simulink subsystem "Final_Project_DistHold_attempt_20260602_205044"  (R2024a)
settings: Solver=VariableStepAuto  StartTime=0.0  StopTime=10.0  RelTol=1e-3
values from neighbouring files (symbols this model uses):
  D = hypot(Ep(:,1)-Tp(:,1)',Ep(:,2)-Tp(:,2)')    [pp_compare_stage.m]    (also in pp_diag_path.m; pp_t09_clear.m = hypot(Ep(:,1)-Tperim(:,1)', Ep(:,2)-Tperim(:,2)'); pp_tune2.m)
undefined symbols (not defined in the file or in its folder): DiscIntNeverNeededParam, waypoint_const
libraries: CarMaker4SL x83, simulink x2
(part 3 of 5)

== matlab function Final_Project_DistHold_attempt_20260602_205044/Driving_Module_Ver.3_PSH/Subsystem/Traffic_Detector ==
  data: ego_state input Bus: EgoStateBus; lead_dist output double; lanes input Bus: ParsedLaneBus; traffic input; target_speed input double; ego_lane_id input int32; lead_speed output double; left_clear output boolean; right_clear output boolean
function [lead_dist, lead_speed, left_clear, right_clear] = Traffic_Detector(ego_state, lanes, traffic, target_speed, ego_lane_id)
%#codegen
% traffic : Obstacle_Info_Bus
% 내부 구조 예:
%   traffic.t16.x, traffic.t16.y, traffic.t16.vx, traffic.t16.vy
%   ...
%   traffic.t28.x, traffic.t28.y, traffic.t28.vx, traffic.t28.vy
%
% 주의:
%   target_speed는 배선 호환용으로 남겨두지만, 거리 판단에는 ego_v를 사용함.

    unused_target_speed = target_speed; %#ok<NASGU>

    % ============================================================
    % 0. 출력 초기화
    % ============================================================
    lead_dist   = 1e9;
    lead_speed  = 0.0;
    left_clear  = true;
    right_clear = true;
    ego_lane    = int32(ego_lane_id);

    % ============================================================
    % 1. Ego unpack
    % ============================================================
    ego_x = ego_state.Car_Fr1_tx;
    ego_y = ego_state.Car_Fr1_ty;
    ego_v = ego_state.Ego_V;

    % ============================================================
    % 2. Lane unpack - 5차선
    % ============================================================
    x1 = lanes.x1; y1 = lanes.y1;
    x2 = lanes.x2; y2 = lanes.y2;
    x3 = lanes.x3; y3 = lanes.y3;
    x4 = lanes.x4; y4 = lanes.y4;
    x5 = lanes.x5; y5 = lanes.y5;

    % detector와 lane5 기준을 맞추기 위한 보정
    L5_OFFSET = 1.0;
    x5 = x5 + L5_OFFSET;

    % ============================================================
    % 3. Ego 속도 기반 가변 탐색/안전거리
    % ============================================================
    v_ego_gap = abs(ego_v);

    if v_ego_gap > 60.0
        v_ego_gap = v_ego_gap / 3.6;
    end

    LOOK_FRONT = calcLookFront(v_ego_gap);

    CLEAR_BACK_MIN = 5.0;
    CLEAR_BACK_TG  = 0.5;
    CLEAR_BACK_MAX = 35.0;

    CLEAR_BACK = CLEAR_BACK_MIN + CLEAR_BACK_TG * v_ego_gap;

    if CLEAR_BACK > CLEAR_BACK_MAX
        CLEAR_BACK = CLEAR_BACK_MAX;
    end

    CLEAR_FRONT_MIN = 15.0;
    CLEAR_FRONT_TG  = 0.9;
    CLEAR_FRONT_MAX = 70.0;

    CLEAR_FRONT = CLEAR_FRONT_MIN + CLEAR_FRONT_TG * v_ego_gap;

    if CLEAR_FRONT > CLEAR_FRONT_MAX
        CLEAR_FRONT = CLEAR_FRONT_MAX;
    end

    % ============================================================
    % 4. Init
    % ============================================================
    lead_dist  = 1e9;
    lead_speed = v_ego_gap;

    left_clear  = true;
    right_clear = true;

    if ego_lane >= int32(5)
        left_clear = false;
    end

    if ego_lane <= int32(1)
        right_clear = false;
    end

    % ============================================================
    % 5. Traffic_Info_16_Bus ~ Traffic_Info_28_Bus 직접 처리
    % ============================================================
    [lead_dist, lead_speed, left_clear, right_clear] = check_one_signal( ...
        traffic.t16.x, traffic.t16.y, traffic.t16.vx, traffic.t16.vy, true, ...
        ego_x, ego_y, ego_lane, ...
        x1,y1,x2,y2,x3,y3,x4,y4,x5,y5, ...
        lead_dist, lead_speed, left_clear, right_clear, ...
        LOOK_FRONT, CLEAR_BACK, CLEAR_FRONT);

    [lead_dist, lead_speed, left_clear, right_clear] = check_one_signal( ...
        traffic.t17.x, traffic.t17.y, traffic.t17.vx, traffic.t17.vy, true, ...
        ego_x, ego_y, ego_lane, ...
        x1,y1,x2,y2,x3,y3,x4,y4,x5,y5, ...
        lead_dist, lead_speed, left_clear, right_clear, ...
        LOOK_FRONT, CLEAR_BACK, CLEAR_FRONT);

    [lead_dist, lead_speed, left_clear, right_clear] = check_one_signal( ...
        traffic.t18.x, traffic.t18.y, traffic.t18.vx, traffic.t18.vy, true, ...
        ego_x, ego_y, ego_lane, ...
        x1,y1,x2,y2,x3,y3,x4,y4,x5,y5, ...
        lead_dist, lead_speed, left_clear, right_clear, ...
        LOOK_FRONT, CLEAR_BACK, CLEAR_FRONT);

    [lead_dist, lead_speed, left_clear, right_clear] = check_one_signal( ...
        traffic.t19.x, traffic.t19.y, traffic.t19.vx, traffic.t19.vy, true, ...
        ego_x, ego_y, ego_lane, ...
        x1,y1,x2,y2,x3,y3,x4,y4,x5,y5, ...
        lead_dist, lead_speed, left_clear, right_clear, ...
        LOOK_FRONT, CLEAR_BACK, CLEAR_FRONT);

    [lead_dist, lead_speed, left_clear, right_clear] = check_one_signal( ...
        traffic.t20.x, traffic.t20.y, traffic.t20.vx, traffic.t20.vy, true, ...
        ego_x, ego_y, ego_lane, ...
        x1,y1,x2,y2,x3,y3,x4,y4,x5,y5, ...
        lead_dist, lead_speed, left_clear, right_clear, ...
        LOOK_FRONT, CLEAR_BACK, CLEAR_FRONT);

    [lead_dist, lead_speed, left_clear, right_clear] = check_one_signal( ...
        traffic.t21.x, traffic.t21.y, traffic.t21.vx, traffic.t21.vy, true, ...
        ego_x, ego_y, ego_lane, ...
        x1,y1,x2,y2,x3,y3,x4,y4,x5,y5, ...
        lead_dist, lead_speed, left_clear, right_clear, ...
        LOOK_FRONT, CLEAR_BACK, CLEAR_FRONT);

    [lead_dist, lead_speed, left_clear, right_clear] = check_one_signal( ...
        traffic.t22.x, traffic.t22.y, traffic.t22.vx, traffic.t22.vy, true, ...
        ego_x, ego_y, ego_lane, ...
        x1,y1,x2,y2,x3,y3,x4,y4,x5,y5, ...
        lead_dist, lead_speed, left_clear, right_clear, ...
        LOOK_FRONT, CLEAR_BACK, CLEAR_FRONT);

    [lead_dist, lead_speed, left_clear, right_clear] = check_one_signal( ...
        traffic.t23.x, traffic.t23.y, traffic.t23.vx, traffic.t23.vy, true, ...
        ego_x, ego_y, ego_lane, ...
        x1,y1,x2,y2,x3,y3,x4,y4,x5,y5, ...
        lead_dist, lead_speed, left_clear, right_clear, ...
        LOOK_FRONT, CLEAR_BACK, CLEAR_FRONT);

    [lead_dist, lead_speed, left_clear, right_clear] = check_one_signal( ...
        traffic.t24.x, traffic.t24.y, traffic.t24.vx, traffic.t24.vy, true, ...
        ego_x, ego_y, ego_lane, ...
        x1,y1,x2,y2,x3,y3,x4,y4,x5,y5, ...
        lead_dist, lead_speed, left_clear, right_clear, ...
        LOOK_FRONT, CLEAR_BACK, CLEAR_FRONT);

    [lead_dist, lead_speed, left_clear, right_clear] = check_one_signal( ...
        traffic.t25.x, traffic.t25.y, traffic.t25.vx, traffic.t25.vy, true, ...
        ego_x, ego_y, ego_lane, ...
        x1,y1,x2,y2,x3,y3,x4,y4,x5,y5, ...
        lead_dist, lead_speed, left_clear, right_clear, ...
        LOOK_FRONT, CLEAR_BACK, CLEAR_FRONT);

    [lead_dist, lead_speed, left_clear, right_clear] = check_one_signal( ...
        traffic.t26.x, traffic.t26.y, traffic.t26.vx, traffic.t26.vy, true, ...
        ego_x, ego_y, ego_lane, ...
        x1,y1,x2,y2,x3,y3,x4,y4,x5,y5, ...
        lead_dist, lead_speed, left_clear, right_clear, ...
        LOOK_FRONT, CLEAR_BACK, CLEAR_FRONT);

    [lead_dist, lead_speed, left_clear, right_clear] = check_one_signal( ...
        traffic.t27.x, traffic.t27.y, traffic.t27.vx, traffic.t27.vy, true, ...
        ego_x, ego_y, ego_lane, ...
        x1,y1,x2,y2,x3,y3,x4,y4,x5,y5, ...
        lead_dist, lead_speed, left_clear, right_clear, ...
        LOOK_FRONT, CLEAR_BACK, CLEAR_FRONT);

    [lead_dist, lead_speed, left_clear, right_clear] = check_one_signal( ...
        traffic.t28.x, traffic.t28.y, traffic.t28.vx, traffic.t28.vy, true, ...
        ego_x, ego_y, ego_lane, ...
        x1,y1,x2,y2,x3,y3,x4,y4,x5,y5, ...
        lead_dist, lead_speed, left_clear, right_clear, ...
        LOOK_FRONT, CLEAR_BACK, CLEAR_FRONT);

end


function LOOK_FRONT = calcLookFront(v)
%#codegen
    v = abs(v);

    if v > 60.0
        v = v / 3.6;
    end

    V_HIGH = 80.0 / 3.6;

    if v < V_HIGH
        LOOK_FRONT = 25.0 + 1.0 * v;
    else
        LOOK_FRONT = 25.0 + 1.0 * V_HIGH + 10.0 * (v - V_HIGH);
    end

    if LOOK_FRONT > 120.0
        LOOK_FRONT = 120.0;
    end
end


function [lead_dist, lead_speed, left_clear, right_clear] = check_one_signal( ...
    obj_x, obj_y, obj_vx, obj_vy, valid, ...
    ego_x, ego_y, ego_lane_id, ...
    x1,y1,x2,y2,x3,y3,x4,y4,x5,y5, ...
    lead_dist, lead_speed, left_clear, right_clear, ...
    LOOK_FRONT, CLEAR_BACK, CLEAR_FRONT)
%#codegen

    if ~valid
        return;
    end

    [lead_dist, lead_speed, left_clear, right_clear] = check_one_vehicle( ...
        ego_x, ego_y, ego_lane_id, ...
        obj_x, obj_y, obj_vx, obj_vy, ...
        x1,y1,x2,y2,x3,y3,x4,y4,x5,y5, ...
        lead_dist, lead_speed, left_clear, right_clear, ...
        LOOK_FRONT, CLEAR_BACK, CLEAR_FRONT);

end


function [lead_dist, lead_speed, left_clear, right_clear] = check_one_vehicle( ...
    ego_x, ego_y, ego_lane_id, ...
    obj_x, obj_y, obj_vx, obj_vy, ...
    x1, y1, x2, y2, x3, y3, x4, y4, x5, y5, ...
    lead_dist, lead_speed, left_clear, right_clear, ...
    LOOK_FRONT, CLEAR_BACK, CLEAR_FRONT)
%#codegen

    [obj_lane_id, obj_idx] = nearest_lane_id( ...
        obj_x, obj_y, ...
        x1, y1, x2, y2, x3, y3, x4, y4, x5, y5);

    if obj_lane_id == ego_lane_id

        ego_idx = nearest_idx_by_lane( ...
            ego_lane_id, ego_x, ego_y, ...
            x1, y1, x2, y2, x3, y3, x4, y4, x5, y5);

        s_rel = arc_dist_forward_by_lane( ...
            ego_lane_id, ego_idx, obj_idx, ...
            x1, y1, x2, y2, x3, y3, x4, y4, x5, y5);

        if s_rel > 0.0 && s_rel < LOOK_FRONT
            if s_rel < lead_dist
                lead_dist  = s_rel;
                lead_speed = sqrt(obj_vx*obj_vx + obj_vy*obj_vy);
            end
        end
    end

    if obj_lane_id == ego_lane_id + int32(1)

        ego_idx_adj = nearest_idx_by_lane( ...
            obj_lane_id, ego_x, ego_y, ...
            x1, y1, x2, y2, x3, y3, x4, y4, x5, y5);

        is_close = is_close_on_adj_lane( ...
            obj_lane_id, ego_idx_adj, obj_idx, ...
            CLEAR_BACK, CLEAR_FRONT, ...
            x1, y1, x2, y2, x3, y3, x4, y4, x5, y5);

        if is_close
            left_clear = false;
        end

    elseif obj_lane_id == ego_lane_id - int32(1)

        ego_idx_adj = nearest_idx_by_lane( ...
            obj_lane_id, ego_x, ego_y, ...
            x1, y1, x2, y2, x3, y3, x4, y4, x5, y5);

        is_close = is_close_on_adj_lane( ...
            obj_lane_id, ego_idx_adj, obj_idx, ...
            CLEAR_BACK, CLEAR_FRONT, ...
            x1, y1, x2, y2, x3, y3, x4, y4, x5, y5);

        if is_close
            right_clear = false;
        end
    end

end


function [lane_id, best_idx] = nearest_lane_id(px, py, x1, y1, x2, y2, x3, y3, x4, y4, x5, y5)
%#codegen

    [idx1, d1] = nearest_idx_d2(x1, y1, px, py);
    [idx2, d2] = nearest_idx_d2(x2, y2, px, py);
    [idx3, d3] = nearest_idx_d2(x3, y3, px, py);
    [idx4, d4] = nearest_idx_d2(x4, y4, px, py);
    [idx5, d5] = nearest_idx_d2(x5, y5, px, py);

    lane_id  = int32(1);
    best_idx = idx1;
    best_d2  = d1;

    if d2 < best_d2
        lane_id  = int32(2);
        best_idx = idx2;
        best_d2  = d2;
    end

    if d3 < best_d2
        lane_id  = int32(3);
        best_idx = idx3;
        best_d2  = d3;
    end

    if d4 < best_d2
        lane_id  = int32(4);
        best_idx = idx4;
        best_d2  = d4;
    end

    if d5 < best_d2
        lane_id  = int32(5);
        best_idx = idx5;
    end

end


function idx = nearest_idx_by_lane(lane_id, px, py, x1, y1, x2, y2, x3, y3, x4, y4, x5, y5)
%#codegen

    if lane_id == int32(1)
        [idx, ~] = nearest_idx_d2(x1, y1, px, py);
    elseif lane_id == int32(2)
        [idx, ~] = nearest_idx_d2(x2, y2, px, py);
    elseif lane_id == int32(3)
        [idx, ~] = nearest_idx_d2(x3, y3, px, py);
    elseif lane_id == int32(4)
        [idx, ~] = nearest_idx_d2(x4, y4, px, py);
    else
        [idx, ~] = nearest_idx_d2(x5, y5, px, py);
    end

end


function [best_i, best_d2] = nearest_idx_d2(xa, ya, px, py)
%#codegen

    best_i  = int32(1);
    best_d2 = 1e12;
    N = int32(numel(xa));

    for i = 1:N
        dx = xa(i) - px;
        dy = ya(i) - py;
        d2 = dx*dx + dy*dy;

        if d2 < best_d2
            best_d2 = d2;
            best_i  = i;
        end
    end

end


function ds = arc_dist_forward_by_lane(lane_id, idx_from, idx_to, ...
    x1, y1, x2, y2, x3, y3, x4, y4, x5, y5)
%#codegen

    if lane_id == int32(1)
        ds = arc_dist_forward_closed(x1, y1, idx_from, idx_to);
    elseif lane_id == int32(2)
        ds = arc_dist_forward_closed(x2, y2, idx_from, idx_to);
    elseif lane_id == int32(3)
        ds = arc_dist_forward_closed(x3, y3, idx_from, idx_to);
    elseif lane_id == int32(4)
        ds = arc_dist_open(x4, y4, idx_from, idx_to);
    else
        ds = arc_dist_open(x5, y5, idx_from, idx_to);
    end

end


function ds = arc_dist_forward_closed(xa, ya, idx_from, idx_to)
%#codegen

    ds = 0.0;
    N = int32(numel(xa));

    if idx_to == idx_from
        ds = 0.0;
        return;
    end

    if idx_to > idx_from

        for i = idx_from:(idx_to - int32(1))
            dx = xa(i+1) - xa(i);
            dy = ya(i+1) - ya(i);
            ds = ds + sqrt(dx*dx + dy*dy);
        end

    else

        for i = idx_from:(N - int32(1))
            dx = xa(i+1) - xa(i);
            dy = ya(i+1) - ya(i);
            ds = ds + sqrt(dx*dx + dy*dy);
        end

        dx = xa(1) - xa(N);
        dy = ya(1) - ya(N);
        ds = ds + sqrt(dx*dx + dy*dy);

        for i = int32(1):(idx_to - int32(1))
            dx = xa(i+1) - xa(i);
            dy = ya(i+1) - ya(i);
            ds = ds + sqrt(dx*dx + dy*dy);
        end

    end

end


function is_close = is_close_on_adj_lane(lane_id, idx_from, idx_to, ...
    CLEAR_BACK, CLEAR_FRONT, ...
    x1, y1, x2, y2, x3, y3, x4, y4, x5, y5)
%#codegen

    is_close = false;

    if lane_id == int32(1)

        fwd_dist  = arc_dist_forward_closed(x1, y1, idx_from, idx_to);
        total_len = arc_length_closed(x1, y1);
        back_dist = total_len - fwd_dist;

        if fwd_dist < CLEAR_FRONT || back_dist < CLEAR_BACK
            is_close = true;
        end

    elseif lane_id == int32(2)

        fwd_dist  = arc_dist_forward_closed(x2, y2, idx_from, idx_to);
        total_len = arc_length_closed(x2, y2);
        back_dist = total_len - fwd_dist;

        if fwd_dist < CLEAR_FRONT || back_dist < CLEAR_BACK
            is_close = true;
        end

    elseif lane_id == int32(3)

        fwd_dist  = arc_dist_forward_closed(x3, y3, idx_from, idx_to);
        total_len = arc_length_closed(x3, y3);
        back_dist = total_len - fwd_dist;

        if fwd_dist < CLEAR_FRONT || back_dist < CLEAR_BACK
            is_close = true;
        end

    elseif lane_id == int32(4)

        s_rel = arc_dist_open(x4, y4, idx_from, idx_to);

        if s_rel > -CLEAR_BACK && s_rel < CLEAR_FRONT
            is_close = true;
        end

    else

        s_rel = arc_dist_open(x5, y5, idx_from, idx_to);

        if s_rel > -CLEAR_BACK && s_rel < CLEAR_FRONT
            is_close = true;
        end

    end

end


function total_len = arc_length_closed(xa, ya)
%#codegen

    total_len = 0.0;
    N = int32(numel(xa));

    for i = int32(1):(N - int32(1))
        dx = xa(i+1) - xa(i);
        dy = ya(i+1) - ya(i);
        total_len = total_len + sqrt(dx*dx + dy*dy);
    end

    dx = xa(1) - xa(N);
    dy = ya(1) - ya(N);
    total_len = total_len + sqrt(dx*dx + dy*dy);

end


function ds = arc_dist_open(xa, ya, idx_from, idx_to)
%#codegen

    ds = 0.0;

    if idx_to == idx_from

        ds = 0.0;

    elseif idx_to > idx_from

        for i = idx_from:(idx_to - int32(1))
            dx = xa(i+1) - xa(i);
            dy = ya(i+1) - ya(i);
            ds = ds + sqrt(dx*dx + dy*dy);
        end

    else

        for i = idx_to:(idx_from - int32(1))
            dx = xa(i+1) - xa(i);
            dy = ya(i+1) - ya(i);
            ds = ds - sqrt(dx*dx + dy*dy);
        end

    end

end

== matlab function Final_Project_DistHold_attempt_20260602_205044/Driving_Module_Ver.3_PSH/Subsystem/Decision ==
  data: ego_cross_track_err input; lead_dist input; left_clear input; right_clear input; submission_state input; desired_lane output int32; ego_state input; drive_state output; lane_settled output; ego_lane_id input
function [desired_lane, drive_state, lane_settled] = Decision(ego_cross_track_err, lead_dist, left_clear, right_clear, submission_state, ego_state, ego_lane_id)
%#codegen

    % ============================================================
    % Parameters
    % ============================================================
    LCHG_TRIG_D     = 25.0;
    LAT_ARRIVED     = 0.5;

    MIN_LANE        = int32(1);
    MAX_NORMAL_LANE = int32(3);
    MAX_LANE        = int32(5);

    MODE_ACC  = int32(0);
    MODE_LCHG = int32(1);
    MODE_PARK = int32(2);

    MIN_LCHG_STEP = int32(120);

    PARK_FRONT_HOLD_D = 8.0;

    % ============================================================
    % Ego position
    % ============================================================
    ego_x = ego_state.Car_Fr1_tx;
    ego_y = ego_state.Car_Fr1_ty;

    % ============================================================
    % Parking entry waypoints
    % ============================================================
    L4_X = -46.856;  L4_Y = 15.842;
    L5_X =  -6.845;  L5_Y = 12.658;

    DIST_PREP_L3  = 150.0;
    DIST_ENTER_L4 = 20.0;
    DIST_ENTER_L5 =  8.0;

    % ============================================================
    % Persistent states
    % ============================================================
    persistent target_lane_p mode_p lchg_timer_p park_state did_init

    if isempty(did_init)
        target_lane_p = int32(2);
        mode_p        = MODE_ACC;
        lchg_timer_p  = int32(0);
        park_state    = int32(0);
        did_init      = true;
    end

    % ============================================================
    % 기본 출력
    % lane_settled은 차선변경 완료 순간에만 true pulse
    % ============================================================
    desired_lane  = target_lane_p;
    drive_state   = mode_p;
    lane_settled  = false;

    % ============================================================
    % Safety clamp
    % ============================================================
    if target_lane_p < MIN_LANE
        target_lane_p = MIN_LANE;
    elseif target_lane_p > MAX_LANE
        target_lane_p = MAX_LANE;
    end

    % ============================================================
    % Distance to parking waypoints
    % ============================================================
    dist_l4 = sqrt((ego_x - L4_X)^2 + (ego_y - L4_Y)^2);
    dist_l5 = sqrt((ego_x - L5_X)^2 + (ego_y - L5_Y)^2);

    % ============================================================
    % Parking command latch
    %
    % 톨게이트 selector가 target_lane을 1차선으로 override했기 때문에
    % decision 내부 target_lane_p와 실제 차량 차선이 다를 수 있음.
    % submission_state가 처음 들어오는 순간 target_lane_p를 ego_lane_id로 동기화.
    % ============================================================
    if park_state == int32(0)
        if submission_state == int32(1)

            target_lane_p = int32(ego_lane_id);

            if target_lane_p < int32(1)
                target_lane_p = int32(1);
            elseif target_lane_p > int32(3)
                target_lane_p = int32(3);
            end

            mode_p       = MODE_ACC;
            lchg_timer_p = int32(0);

            park_state = int32(1);
        end
    end

    % ============================================================
    % 주차장 진입 중 새 차선변경 시작 가능 여부
    % ============================================================
    front_ok_for_new_lchg = true;

    if lead_dist < PARK_FRONT_HOLD_D
        front_ok_for_new_lchg = false;
    end

    % ============================================================
    % Parking state machine
    % ============================================================
    if park_state == int32(1)

        if mode_p ~= MODE_LCHG && ...
           dist_l4 < DIST_PREP_L3 && ...
           target_lane_p ~= int32(3) && ...
           front_ok_for_new_lchg

            next_lane = target_lane_p;

            if target_lane_p < int32(3)
                next_lane = target_lane_p + int32(1);
            elseif target_lane_p > int32(3)
                next_lane = target_lane_p - int32(1);
            end

            if can_change_one_lane(target_lane_p, next_lane, left_clear, right_clear)

                target_lane_p = next_lane;
                mode_p        = MODE_LCHG;
                lchg_timer_p  = MIN_LCHG_STEP;

            end
        end

        if mode_p ~= MODE_LCHG && ...
           dist_l4 < DIST_ENTER_L4 && ...
           target_lane_p == int32(3) && ...
           front_ok_for_new_lchg

            next_lane = int32(4);

            if can_change_one_lane(target_lane_p, next_lane, left_clear, right_clear)

                target_lane_p = next_lane;
                mode_p        = MODE_LCHG;
                lchg_timer_p  = MIN_LCHG_STEP;
                park_state    = int32(2);

            end
        end

    elseif park_state == int32(2)

        if target_lane_p == int32(4) && mode_p ~= MODE_LCHG
            park_state = int32(3);
        end

    elseif park_state == int32(3)

        if mode_p ~= MODE_LCHG && ...
           dist_l5 < DIST_ENTER_L5 && ...
           front_ok_for_new_lchg

            next_lane = int32(5);

            if can_change_one_lane(target_lane_p, next_lane, left_clear, right_clear)

                target_lane_p = next_lane;
                mode_p        = MODE_LCHG;
                lchg_timer_p  = MIN_LCHG_STEP;
                park_state    = int32(4);

            end
        end

    elseif park_state == int32(4)

        if target_lane_p == int32(5) && mode_p ~= MODE_LCHG
            mode_p     = MODE_PARK;
            park_state = int32(5);
        end

    elseif park_state >= int32(5)

        mode_p = MODE_PARK;
    end

    % ============================================================
    % Parking 진행 중이면 일반 주행 로직을 타지 않음
    % ============================================================
    if park_state > int32(0)

        if mode_p == MODE_LCHG

            if lchg_timer_p > int32(0)

                lchg_timer_p = lchg_timer_p - int32(1);

            else

                if abs(ego_cross_track_err) < LAT_ARRIVED
                    mode_p       = MODE_ACC;
                    lane_settled = true;
                end

            end
        end

        desired_lane = target_lane_p;
        drive_state  = mode_p;
        return;
    end

    % ============================================================
    % 일반 주행 로직
    % ============================================================
    if mode_p == MODE_ACC

        if lead_dist < LCHG_TRIG_D

            if left_clear && target_lane_p < MAX_NORMAL_LANE

                target_lane_p = target_lane_p + int32(1);
                mode_p        = MODE_LCHG;
                lchg_timer_p  = MIN_LCHG_STEP;

            elseif right_clear && target_lane_p > MIN_LANE

                target_lane_p = target_lane_p - int32(1);
                mode_p        = MODE_LCHG;
                lchg_timer_p  = MIN_LCHG_STEP;

            end
        end

    else

        if lchg_timer_p > int32(0)

            lchg_timer_p = lchg_timer_p - int32(1);

        else

            if abs(ego_cross_track_err) < LAT_ARRIVED

                mode_p       = MODE_ACC;
                lane_settled = true;

            end
        end
    end

    % ============================================================
    % 갱신된 출력
    % ============================================================
    desired_lane = target_lane_p;
    drive_state  = mode_p;

end


function ok = can_change_one_lane(cur_lane, next_lane, left_clear, right_clear)
%#codegen

    ok = false;

    if next_lane == cur_lane

        ok = true;

    elseif next_lane == cur_lane + int32(1)

        if left_clear
            ok = true;
        end

    elseif next_lane == cur_lane - int32(1)

        if right_clear
            ok = true;
        end

    else

        ok = false;

    end

end

== matlab function Final_Project_DistHold_attempt_20260602_205044/Driving_Module_Ver.3_PSH/Subsystem/Tollgate_Selector ==
  data: ego_state input; target_lane_out output; tollgate_cmd input; desired_lane input; ego_lane_id input; ego_cross_track_err input; ego_max_curvature input; left_clear input; right_clear input; toll_speed_limit output; toll_target_lane_cmd input; toll_pass_speed_cmd input
function [target_lane_out, toll_speed_limit] = tollgate_selector( ...
    ego_state, tollgate_cmd, desired_lane, ego_lane_id, ego_cross_track_err, ego_max_curvature, left_clear, right_clear, ...
    toll_target_lane_cmd, toll_pass_speed_cmd)
%#codegen

    % ============================================================
    % Cmd 정의
    % 0 : Default
    % 1 : Parking
    % 2 : Tollgate
    % ============================================================
    CMD_TOLLGATE = int32(2);

    % ============================================================
    % 지정 톨게이트 차선
    % 외부 입력으로 받음
    % ============================================================
    TOLL_TARGET_LANE = int32(toll_target_lane_cmd);

    % ============================================================
    % 톨게이트 좌표
    % ============================================================
    G1_X = -176.212;
    G1_Y = -86.9523;

    G2_X = -172.724;
    G2_Y = -86.2036;

    G3_X = -169.207;
    G3_Y = -87.124;

    % ============================================================
    % 거리 / 속도 파라미터
    % ============================================================
    TOLL_REACHED_DIST = 6.0;
    SPEED_NONE        = 1.0e9;

    TOLL_APPROACH_SPEED = 50.0 / 3.6;
    TOLL_GAP_SPEED      = 30.0 / 3.6;
    TOLL_CRAWL_SPEED    = 5.0  / 3.6;
    TOLL_PASS_SPEED     = toll_pass_speed_cmd;

    % toll_pass_speed_cmd가 km/h로 들어오는 경우 보호
    if TOLL_PASS_SPEED > 20.0
        TOLL_PASS_SPEED = TOLL_PASS_SPEED / 3.6;
    end

    TOLL_APPROACH_DIST  = 100.0;

    LANE_CHANGE_DIST = 45.0;
    DIST_MARGIN      = 20.0;

    % ============================================================
    % 한 차선 이동 후 안정 판단
    % ============================================================
    LAT_SETTLE    = 0.6;
    MIN_HOLD_STEP = int32(80);    % 0.01초 기준 0.8초

    % ============================================================
    % 톨게이트 모드 진입 직후 대기
    % ============================================================
    ENTER_WAIT_STEP = int32(30);  % 0.01초 기준 0.3초 대기

    % ============================================================
    % 고속/커브 상황에서 차선변경 시작 억제
    % ============================================================
    LCHG_START_MAX_V = 55.0 / 3.6;
    CURVE_START_MAX  = 0.018;
    LOW_SPEED_ALLOW  = 35.0 / 3.6;

    % ============================================================
    % Ego unpack
    % ============================================================
    ego_x = ego_state.Car_Fr1_tx;
    ego_y = ego_state.Car_Fr1_ty;
    ego_v = ego_state.Ego_V;

    % ============================================================
    % persistent 상태
    % passed_p : 내부 톨게이트 통과 상태
    % ============================================================
    persistent passed_p prev_toll_p step_lane_p hold_count_p enter_wait_p did_init

    if isempty(did_init)
        passed_p     = false;
        prev_toll_p  = false;
        step_lane_p  = int32(2);
        hold_count_p = int32(0);
        enter_wait_p = int32(0);
        did_init     = true;
    end

    % ============================================================
    % 기본 출력
    % desired_lane은 parking 모드에서 4 또는 5가 될 수 있으므로
    % 여기서는 기본값을 절대 1~3으로 clamp하면 안 됨.
    % ============================================================
    target_lane_out  = int32(desired_lane);
    toll_speed_limit = SPEED_NONE;

    toll_now = (int32(tollgate_cmd) == CMD_TOLLGATE);

    % ============================================================
    % tollgate_cmd가 2로 처음 들어오는 순간 초기화
    % ============================================================
    if toll_now && ~prev_toll_p
        passed_p = false;

        % 진입 순간에는 기존 desired_lane을 유지
        step_lane_p  = clamp_toll_lane(desired_lane);
        hold_count_p = int32(0);
        enter_wait_p = ENTER_WAIT_STEP;
    end

    prev_toll_p = toll_now;

    % ============================================================
    % tollgate_cmd가 2가 아니면 톨게이트 개입 없음
    % ============================================================
    if ~toll_now
        passed_p         = false;
        toll_speed_limit = SPEED_NONE;

        hold_count_p     = int32(0);
        enter_wait_p     = int32(0);
        target_lane_out  = int32(desired_lane);
        return;
    end

    % ============================================================
    % 이미 톨게이트 통과 후인 경우
    % ============================================================
    if passed_p
        target_lane_out  = TOLL_TARGET_LANE;
        toll_speed_limit = SPEED_NONE;
        return;
    end

    % ============================================================
    % 선택된 톨게이트 좌표
    % ============================================================
    if TOLL_TARGET_LANE == int32(1)
        gate_x = G1_X;
        gate_y = G1_Y;
    elseif TOLL_TARGET_LANE == int32(2)
        gate_x = G2_X;
        gate_y = G2_Y;
    else
        gate_x = G3_X;
        gate_y = G3_Y;
    end

    % ============================================================
    % 톨게이트까지 거리
    % ============================================================
    dx = ego_x - gate_x;
    dy = ego_y - gate_y;
    dist_to_toll = sqrt(dx * dx + dy * dy);

    % ============================================================
    % 현재 차선 / 중간 목표 차선 정리
    % ============================================================
    current_lane = clamp_toll_lane(ego_lane_id);
    step_lane_p  = clamp_toll_lane(step_lane_p);

    % ============================================================
    % 속도 단위 방어
    % ============================================================
    v = ego_v;

    if v > 60.0
        v = v / 3.6;
    end

    % ============================================================
    % 고속/커브 차선변경 시작 조건
    % ============================================================
    speed_ok = (v <= LCHG_START_MAX_V);

    if ego_max_curvature <= CURVE_START_MAX
        curve_ok = true;
    elseif v <= LOW_SPEED_ALLOW
        curve_ok = true;
    else
        curve_ok = false;
    end

    start_lchg_ok = speed_ok && curve_ok;

    % ============================================================
    % 톨게이트 모드 진입 직후 보호 구간
    % ============================================================
    if enter_wait_p > int32(0)

        enter_wait_p = enter_wait_p - int32(1);

        target_lane_out  = int32(desired_lane);
        toll_speed_limit = SPEED_NONE;

        if ~speed_ok
            toll_speed_limit = TOLL_APPROACH_SPEED;
        end

        if ~curve_ok
            toll_speed_limit = TOLL_APPROACH_SPEED;
        end

        if dist_to_toll < TOLL_APPROACH_DIST
            if toll_speed_limit > TOLL_APPROACH_SPEED
                toll_speed_limit = TOLL_APPROACH_SPEED;
            end
        end

        if enter_wait_p == int32(0)
            step_lane_p  = current_lane;
            hold_count_p = int32(0);
        end

        return;
    end

    % ============================================================
    % 옆차선 clear 확인
    % ============================================================
    if step_lane_p > TOLL_TARGET_LANE
        side_clear_ok = (right_clear ~= 0);
    elseif step_lane_p < TOLL_TARGET_LANE
        side_clear_ok = (left_clear ~= 0);
    else
        side_clear_ok = true;
    end

    % ============================================================
    % Mandatory tollgate 속도 제한
    % ============================================================
    lanes_remaining = abs(double(current_lane) - double(TOLL_TARGET_LANE));

    if lanes_remaining > 0.0

        required_dist = lanes_remaining * LANE_CHANGE_DIST + DIST_MARGIN;

        toll_speed_limit = SPEED_NONE;

        if ~speed_ok
            toll_speed_limit = TOLL_APPROACH_SPEED;
        end

        if ~curve_ok
            toll_speed_limit = TOLL_APPROACH_SPEED;
        end

        if ~side_clear_ok
            toll_speed_limit = TOLL_GAP_SPEED;
        end

        if dist_to_toll < required_dist
            toll_speed_limit = TOLL_CRAWL_SPEED;
        end

    else

        if dist_to_toll < TOLL_APPROACH_DIST
            toll_speed_limit = TOLL_PASS_SPEED;
        else
            toll_speed_limit = SPEED_NONE;
        end
    end

    % ============================================================
    % 한 차선씩만 이동
    % ============================================================
    if step_lane_p ~= TOLL_TARGET_LANE

        if current_lane == step_lane_p

            if abs(ego_cross_track_err) < LAT_SETTLE
                hold_count_p = hold_count_p + int32(1);
            else
                hold_count_p = int32(0);
            end

            if hold_count_p >= MIN_HOLD_STEP && start_lchg_ok && side_clear_ok

                if step_lane_p < TOLL_TARGET_LANE
                    step_lane_p = step_lane_p + int32(1);
                elseif step_lane_p > TOLL_TARGET_LANE
                    step_lane_p = step_lane_p - int32(1);
                end

                step_lane_p  = clamp_toll_lane(step_lane_p);
                hold_count_p = int32(0);
            end

        else
            hold_count_p = int32(0);
        end
    end

    % ============================================================
    % 최종 출력 target_lane
    % ============================================================
    target_lane_out = step_lane_p;

    % ============================================================
    % 톨게이트 통과 판단
    % ============================================================
    if dist_to_toll < TOLL_REACHED_DIST
        passed_p = true;

        target_lane_out  = TOLL_TARGET_LANE;
        toll_speed_limit = SPEED_NONE;
    end

end


function lane = clamp_toll_lane(lane_in)
%#codegen
    lane = int32(lane_in);

    if lane < int32(1)
        lane = int32(1);
    elseif lane > int32(3)
        lane = int32(3);
    end
end

== matlab function Final_Project_DistHold_attempt_20260602_205044/Driving_Module_Ver.3_PSH/Subsystem/Controller ==
  data: ego_cross_track_err input; steer output; ego_head_err input; ego_max_curvature input; target_speed input; lead_dist input; lead_speed input; drive_state input; lane_settled input; submission_state input; ego_state input; accel output; front_dist_lock output; gear_pos output
function [steer, accel, front_dist_lock, gear_pos] = controller(...
    ego_cross_track_err, ego_head_err, ego_max_curvature, target_speed, ...
    lead_dist, lead_speed, drive_state, lane_settled, submission_state, ego_state)
%#codegen

    % ============================================================
    % 기본 상수
    % ============================================================
    TS           = 0.01;
    STEER_LIM    = 0.58;
    MAX_SPEED    = 50.0;
    MODE_LCHG    = int32(1);
    MODE_PARK    = int32(2);
    KAPPA_EPS    = 1e-4;
    SPD_DEADBAND = 0.3;

    % ============================================================
    % Ego unpack
    % ============================================================
    ego_x = ego_state.Car_Fr1_tx;
    ego_y = ego_state.Car_Fr1_ty;
    ego_v = ego_state.Ego_V;

    % ============================================================
    % Parking waypoints
    % ============================================================
    L4_X     = -46.856;  L4_Y     = 15.842;
    L5_END_X =  2.617;   L5_END_Y = -35.0;

    dist_l4     = sqrt((ego_x - L4_X)^2     + (ego_y - L4_Y)^2);
    dist_to_end = sqrt((ego_x - L5_END_X)^2 + (ego_y - L5_END_Y)^2);

    % ============================================================
    % 파라미터 정의: 일반 주행 / 주차 진입
    % ============================================================
    K_STANLEY_NRM  = 0.88;   K_STANLEY_PRK  = 0.20;
    KP_HEAD_NRM    = 0.90;   KP_HEAD_PRK    = 0.50;
    LOOK_FRONT_NRM = calcLookFront(ego_v);  LOOK_FRONT_PRK = 10.0;
    ALAT_NRM       = 3.50;   ALAT_PRK       = 1.50;
    ATOT_NRM       = 4.00;   ATOT_PRK       = 2.00;
    MCSPD_NRM      = 7.00;   MCSPD_PRK      = 1.00;
    VREF_A_NRM     = 50.0;   VREF_A_PRK     = 2.00;
    VREF_D_NRM     = 100.0;  VREF_D_PRK     = 5.00;
    JERK_U_NRM     = 50.0;   JERK_U_PRK     = 3.00;
    JERK_D_NRM     = 60.0;   JERK_D_PRK     = 5.00;
    AMAX_NRM       = 10.0;   AMAX_PRK       = 3.00;
    DMAX_NRM       = 10.0;   DMAX_PRK       = 5.00;

    % ============================================================
    % park_cmd에 따른 파라미터 보간
    % L4에 가까워질수록 일반 주행 -> 주차 진입 파라미터로 전환
    % ============================================================
    FADE_FAR  = 50.0;
    FADE_NEAR = 20.0;

    if submission_state == int32(1)
        if dist_l4 >= FADE_FAR
            r = 0.0;
        elseif dist_l4 <= FADE_NEAR
            r = 1.0;
        else
            r = (FADE_FAR - dist_l4) / (FADE_FAR - FADE_NEAR);
        end
    else
        r = 0.0;
    end

    K_STANLEY       = K_STANLEY_NRM  + r * (K_STANLEY_PRK  - K_STANLEY_NRM);
    KP_HEAD         = KP_HEAD_NRM    + r * (KP_HEAD_PRK    - KP_HEAD_NRM);
    LOOK_FRONT      = LOOK_FRONT_NRM + r * (LOOK_FRONT_PRK - LOOK_FRONT_NRM);
    A_LAT_LIMIT     = ALAT_NRM       + r * (ALAT_PRK       - ALAT_NRM);
    A_TOTAL_LIMIT   = ATOT_NRM       + r * (ATOT_PRK       - ATOT_NRM);
    MIN_CURVE_SPEED = MCSPD_NRM      + r * (MCSPD_PRK      - MCSPD_NRM);
    V_REF_ACCEL     = VREF_A_NRM     + r * (VREF_A_PRK     - VREF_A_NRM);
    V_REF_DECEL     = VREF_D_NRM     + r * (VREF_D_PRK     - VREF_D_NRM);
    JERK_UP         = JERK_U_NRM     + r * (JERK_U_PRK     - JERK_U_NRM);
    JERK_DOWN       = JERK_D_NRM     + r * (JERK_D_PRK     - JERK_D_NRM);
    ACCEL_MAX_BASE  = AMAX_NRM       + r * (AMAX_PRK       - AMAX_NRM);
    DECEL_MAX_BASE  = DMAX_NRM       + r * (DMAX_PRK       - DMAX_NRM);

    % ============================================================
    % L4 통과 latch
    % ============================================================
    persistent l4_passed_p l4_pass_init_p

    if isempty(l4_pass_init_p)
        l4_passed_p    = false;
        l4_pass_init_p = true;
    end

    if submission_state ~= int32(1)
        l4_passed_p = false;
    end

    L4_PASS_DIST = 3.0;

    if submission_state == int32(1) && dist_l4 < L4_PASS_DIST
        l4_passed_p = true;
    end

    % ============================================================
    % 목표속도 결정
    % ============================================================
    if submission_state == int32(1)

        DECEL_DIST = 25.0;
        STOP_DIST  =  2.0;

        SPD_BEFORE_L4_FAR  = 12.3;
        SPD_BEFORE_L4_NEAR = 4.8;
        SPD_AFTER_L4       = 5.8;
        SPD_PARK_INSIDE    = 4.2;

        if drive_state == MODE_PARK

            if dist_to_end < STOP_DIST
                ts = 0.0;
            elseif dist_to_end < DECEL_DIST
                ts = SPD_PARK_INSIDE * (dist_to_end / DECEL_DIST);
            else
                ts = SPD_PARK_INSIDE;
            end

        elseif l4_passed_p

            ts = SPD_AFTER_L4;

        elseif dist_l4 > FADE_NEAR

            if dist_l4 >= FADE_FAR
                ts = SPD_BEFORE_L4_FAR;
            else
                ts = SPD_BEFORE_L4_FAR + ...
                     (SPD_BEFORE_L4_NEAR - SPD_BEFORE_L4_FAR) * r;
            end

        else

            ts = SPD_AFTER_L4;

        end

    else

        ts = target_speed;

        if ts > 20.0
            ts = ts / 3.6;
        end

    end

    if ts > MAX_SPEED
        ts = MAX_SPEED;
    end

    if ts < 0.0
        ts = 0.0;
    end

    % ============================================================
    % persistent
    % ============================================================
    persistent desired_v_p accel_p did_init

    if isempty(did_init)
        desired_v_p = ego_v;
        accel_p     = 0.0;
        did_init    = true;
    end

    % ============================================================
    % 1. Stanley 조향
    % ============================================================
    v_safe = ego_v;

    if v_safe < 1.0
        v_safe = 1.0;
    end

    steer = KP_HEAD * ego_head_err - atan2(K_STANLEY * ego_cross_track_err, v_safe);

    if steer > STEER_LIM
        steer = STEER_LIM;
    elseif steer < -STEER_LIM
        steer = -STEER_LIM;
    end

    % ============================================================
    % 1-1. 끝점 추가 좌회전 블렌드
    % submission_state=1, MODE_PARK, 끝점 5m 이내에서만 적용
    % ============================================================
    EXTRA_DIST = 5.0;
    EXTRA_RAD  = pi / 3.0;

    if submission_state == int32(1) && drive_state == MODE_PARK
        if dist_to_end < EXTRA_DIST && dist_to_end > 0.0
            blend = 1.0 - (dist_to_end / EXTRA_DIST);
            steer = steer + blend * EXTRA_RAD;

            if steer > EXTRA_RAD
                steer = EXTRA_RAD;
            elseif steer < -EXTRA_RAD
                steer = -EXTRA_RAD;
            end
        end
    end

    % ============================================================
    % 2. 곡률 기반 목표속도 제한
    % ============================================================
    desired_v_raw = ts;

    if ego_max_curvature > KAPPA_EPS

        v_curve = sqrt(A_LAT_LIMIT / ego_max_curvature);

        if v_curve < MIN_CURVE_SPEED
            v_curve = MIN_CURVE_SPEED;
        end

        if v_curve < desired_v_raw
            desired_v_raw = v_curve;
        end
    end

    % ============================================================
    % 3. ACC 앞차 감속
    % MODE_PARK 전까지는 앞차 감속 적용
    % ============================================================
    if drive_state ~= MODE_PARK

        if lead_dist < LOOK_FRONT

            time_gap = 2.0;
            ACC_GAIN = 0.5;

            safe_v = lead_speed + (lead_dist - time_gap * ego_v) * ACC_GAIN;

            if safe_v < desired_v_raw
                desired_v_raw = safe_v;
            end
        end
    end

    if desired_v_raw < 0.0
        desired_v_raw = 0.0;
    end

    % ============================================================
    % 4. 목표속도 변화율 제한
    % ============================================================
    dv = desired_v_raw - desired_v_p;

    max_dv_up = V_REF_ACCEL * TS;
    max_dv_dn = V_REF_DECEL * TS;

    if dv > max_dv_up
        desired_v_p = desired_v_p + max_dv_up;
    elseif dv < -max_dv_dn
        desired_v_p = desired_v_p - max_dv_dn;
    else
        desired_v_p = desired_v_raw;
    end

    desired_v = desired_v_p;

    % ============================================================
    % 5. 가감속
    % 주차 구간: 비례제어
    % 일반 구간: 기록 단축용 Bang-Bang
    % ============================================================
    spd_err = desired_v - ego_v;

    if submission_state == int32(1)

        KP_SPD = 2.0;
        accel_cmd = KP_SPD * spd_err;

        if accel_cmd > ACCEL_MAX_BASE
            accel_cmd = ACCEL_MAX_BASE;
        elseif accel_cmd < -DECEL_MAX_BASE
            accel_cmd = -DECEL_MAX_BASE;
        end

    else

        if spd_err > SPD_DEADBAND
            accel_cmd = ACCEL_MAX_BASE;
        elseif spd_err < -SPD_DEADBAND
            accel_cmd = -DECEL_MAX_BASE;
        else
            accel_cmd = 0.5 * spd_err;
        end

    end

    % ============================================================
    % 6. Friction circle 기반 가속 한계
    % ============================================================
    a_lat_now = ego_v * ego_v * ego_max_curvature;

    if a_lat_now >= A_TOTAL_LIMIT
        a_lon_avail = 0.5;
    else
        a_lon_avail = sqrt(A_TOTAL_LIMIT * A_TOTAL_LIMIT - a_lat_now * a_lat_now);

        if a_lon_avail < 0.5
            a_lon_avail = 0.5;
        end
    end

    accel_max = ACCEL_MAX_BASE;

    if a_lon_avail < accel_max
        accel_max = a_lon_avail;
    end

    if accel_cmd > accel_max
        accel_cmd = accel_max;
    end

    if accel_cmd < -DECEL_MAX_BASE
        accel_cmd = -DECEL_MAX_BASE;
    end

    % ============================================================
    % 7. Jerk 제한
    % ============================================================
    da = accel_cmd - accel_p;

    max_da_up = JERK_UP   * TS;
    max_da_dn = JERK_DOWN * TS;

    if da > max_da_up
        accel_p = accel_p + max_da_up;
    elseif da < -max_da_dn
        accel_p = accel_p - max_da_dn;
    else
        accel_p = accel_cmd;
    end

    accel = accel_p;

    % ============================================================
    % 8. front_dist_lock
    % ============================================================
    if drive_state == MODE_LCHG || lane_settled
        front_dist_lock = 0;
    else
        front_dist_lock = lead_dist;
    end

    % ============================================================
    % 9. Gear Position
    % 1 : Drive
    % ============================================================
    gear_pos = int32(1);

end


function LOOK_FRONT = calcLookFront(v)
%#codegen

    v = abs(v);

    if v > 60.0
        v = v / 3.6;
    end

    V_HIGH = 80.0 / 3.6;

    if v < V_HIGH
        LOOK_FRONT = 25.0 + 1.0 * v;
    else
        LOOK_FRONT = 50.0 + 1.0 * V_HIGH + 30.0 * (v - V_HIGH);
    end

    if LOOK_FRONT > 120.0
        LOOK_FRONT = 120.0;
    end

end

== matlab function Final_Project_DistHold_attempt_20260602_205044/Module_Selector/parking_entry_selector ==
  data: parking_map input; module_select output; parking_goal input; parking_start input; ego_global_pos input; waypoints input
function module_select = parking_entry_selector(parking_map, parking_goal, parking_start, ego_global_pos, waypoints) %#codegen
% Module_Selector 상태 (출력 module_select):
%   0 = Driving, 1 = Parking(도달 시 래치 고정), 2 = Tollgate(구간), 3 = 주차목표 도달(래치 고정)
%   톨게이트: (-94.9269,-159.103) 도달 -> 2,  (-172.724,-86.2036) 통과 -> 0
%   주차    : (-141.562,-17.5155) 도달 -> 1 로 래치
%   주차목표: (-2.92924, 9.6997) 도달 -> 3 으로 래치 (최우선)
%   ego_global_pos = [x; y] (Bus Selector+Mux)

persistent parking_latched tollgate_active goal_latched
if isempty(parking_latched)
    parking_latched = false;
end
if isempty(tollgate_active)
    tollgate_active = false;
end
if isempty(goal_latched)
    goal_latched = false;
end

TG_START = [-94.9269, -159.103];   % 톨게이트 시작
TG_END   = [-172.724,  -86.2036];  % 톨게이트 끝
PARK_REF = [-141.562,  -17.5155];  % 주차 진입
GOAL_REF = [-2.92924,    9.6997];  % 주차 목표 지점 (state 3)
R = 6.0;                           % 도달 인정 반경 [m] (자차가 ~5m 옆으로 지나가서 키움)
R_GOAL = 3.0;                      % 주차 목표 도달 반경 [m] (진입로 라인과 구분되도록 작게)

ex = ego_global_pos(1);
ey = ego_global_pos(2);

if hypot(ex - TG_START(1), ey - TG_START(2)) <= R
    tollgate_active = true;
end
if hypot(ex - TG_END(1), ey - TG_END(2)) <= R
    tollgate_active = false;
end

if hypot(ex - PARK_REF(1), ey - PARK_REF(2)) <= R
    parking_latched = true;
end

if hypot(ex - GOAL_REF(1), ey - GOAL_REF(2)) <= R_GOAL
    goal_latched = true;
end

if goal_latched
    module_select = 3.0;
elseif parking_latched
    module_select = 1.0;
elseif tollgate_active
    module_select = 2.0;
else
    module_select = 0.0;
end
end

== stateflow chart Final_Project_DistHold_attempt_20260602_205044/FcnRouter_State ==
  (default) -> (junction 5)
  (junction 5) -> (junction 7) [order 1] : [isPark]{call_park;}
  (junction 5) -> (junction 8) [order 2] : [isPark == 0]{call_drive;}
  data: isPark input double
  events: tick input FUNCTION_CALL_EVENT; call_drive output FUNCTION_CALL_EVENT; call_park output FUNCTION_CALL_EVENT
